simulink model "ev3 robot dynamics simulation"  (R2021a)
settings: Solver=VariableStepAuto  StartTime=0.0  StopTime=10.0  RelTol=1e-3
settings Model: Creator=sanch  LastModifiedBy=hritw
settings SolverCC: AlgebraicLoopSolver=TrustRegion
settings DebuggingCC: SFMachineParentedDataDiag=warning

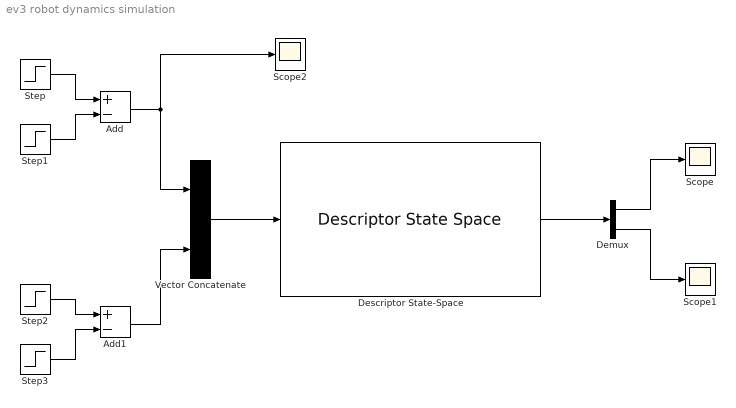
== system ev3 robot dynamics simulation ==
  Add : Sum  Inputs=+-
  Add1 : Sum  Inputs=+-
  Demux : Demux  Outputs=2
  Descriptor State-Space : DescriptorStateSpace  E=[1 0;0 1]  A=[-2.2422 0;0 -2.1672]  B=[.3382 .3382;1.2219 -1.2219]  C=[1 0;0 1]  D=[0 0;0 0]  InitialCondition=[0;0]
  Scope : Scope
  Scope1 : Scope
  Scope2 : Scope
  Step : Step  Time=0  After=3  SampleTime=0
  Step1 : Step  Time=4  After=3  SampleTime=0
  Step2 : Step  Time=0  After=5  SampleTime=0
  Step3 : Step  Time=4  After=5  SampleTime=0
  Vector Concatenate : Concatenate
  wires:
  Vector Concatenate/1 -> Descriptor State-Space/1
  Descriptor State-Space/1 -> Demux/1
  Step/1 -> Add/1
  Step1/1 -> Add/2
  Add/1 -> Vector Concatenate/1, Scope2/1
  Step2/1 -> Add1/1
  Add1/1 -> Vector Concatenate/2
  Step3/1 -> Add1/2
  Demux/2 -> Scope1/1
  Demux/1 -> Scope/1
